simulink model "LADRC_Control"  (R2022a)
settings: Solver=VariableStepAuto  StartTime=0.0  StopTime=20  RelTol=1e-3
undefined symbols (not defined in the file or in its folder): b1, b2, wc, wo
libraries: slpidlib x1
settings Model: Creator=45489  LastModifiedBy=45489
settings SolverCC: AlgebraicLoopSolver=TrustRegion
settings DebuggingCC: UnconnectedInputMsg=warning  UnconnectedOutputMsg=warning  UnconnectedLineMsg=warning  SFMachineParentedDataDiag=warning

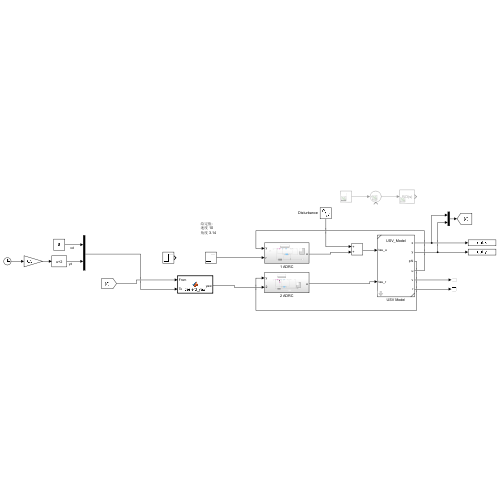
[thumbnail: Simulink's stored preview of the top-level diagram]
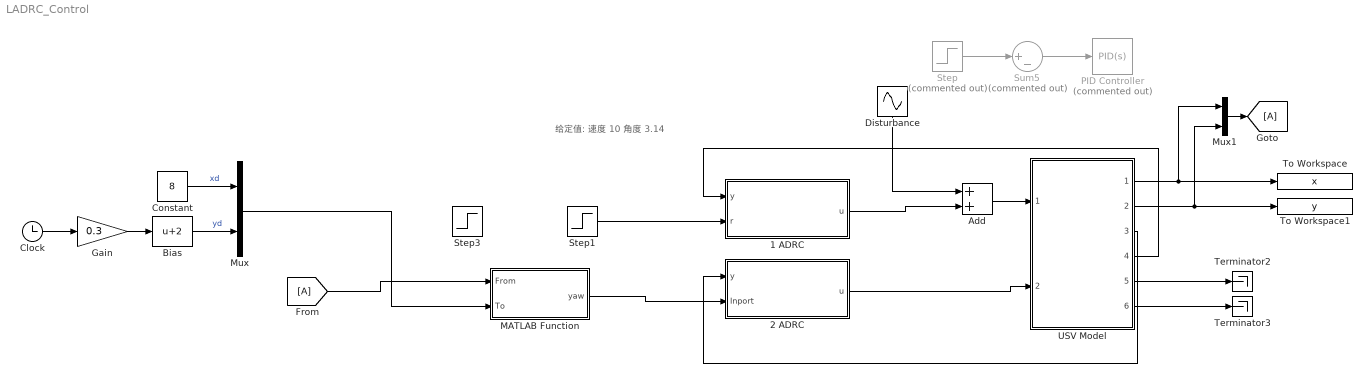
== system LADRC_Control ==
  note: 给定值:
      | 速度 10
      | 角度 3.14
  1 ADRC : Subsystem
  2 ADRC : Subsystem
  Add : Sum
  Bias : Bias  Bias=2  SaturateOnIntegerOverflow=off
  Clock : Clock
  Constant : Constant  Value=8
  Disturbance : Sin  Amplitude=5  Bias=1  SampleTime=0
  From : From
  Gain : Gain  Gain=0.3
  Goto : Goto
  MATLAB Function : MATLAB Function  TreatAsAtomicUnit=on
  Mux : Mux  Inputs=2
  Mux1 : Mux  Inputs=2
  PID Controller : slpidlib/PID Controller  Commented=on  Controller=PID  Form=Parallel  TimeDomain=Continuous-time  UseExternalTs=off  SampleTime=-1  IntegratorMethod=Forward Euler  FilterMethod=Forward Euler  ControllerParametersSource=internal  P=2  I=0  UseKiTs=off  D=1  N=100  UseFilter=on  TunerSelectOption=Transfer Function Based (PID Tuner App)  InitialConditionSource=internal  InitialConditionForIntegrator=0  InitialConditionForFilter=0  DifferentiatorICPrevScaledInput=0  ExternalReset=none  TrackingMode=off  Kt=1  LimitOutput=off  SatLimitsSource=internal  UpperSaturationLimit=inf  LowerSaturationLimit=-inf  LinearizeAsGain=on  AntiWindupMode=none  Kb=1  POutMin=[]  POutMax=[]  IOutMin=[]  IOutMax=[]  DOutMin=[]  DOutMax=[]  NOutMin=[]  NOutMax=[]  SumOutMin=[]  SumOutMax=[]  SaturationOutMin=[]  SaturationOutMax=[]  PParamMin=[]  PParamMax=[]  IParamMin=[]  IParamMax=[]  DParamMin=[]  DParamMax=[]  NParamMin=[]  NParamMax=[]  KbParamMin=[]  KbParamMax=[]  KtParamMin=[]  KtParamMax=[]  KbOutMin=[]  KbOutMax=[]  KtOutMin=[]  KtOutMax=[]  IntegratorOutMin=[]  IntegratorOutMax=[]  FilterOutMin=[]  FilterOutMax=[]  SumI1OutMin=[]  SumI1OutMax=[]  SumI2OutMin=[]  SumI2OutMax=[]  SumI3OutMin=[]  SumI3OutMax=[]  SumI4OutMin=[]  SumI4OutMax=[]  SumDOutMin=[]  SumDOutMax=[]  DifferentiatorOutMin=[]  DifferentiatorOutMax=[]  FilterDiffOutCoefMin=[]  FilterDiffOutCoefMax=[]  ReciprocalOutMin=[]  ReciprocalOutMax=[]  SumDenOutMin=[]  SumDenOutMax=[]  SumNumOutMin=[]  SumNumOutMax=[]  DivideOutMin=[]  DivideOutMax=[]  UdiffTsProdOutMin=[]  UdiffTsProdOutMax=[]  NTsProdOutMin=[]  NTsProdOutMax=[]  UintegralTsProdOutMin=[]  UintegralTsProdOutMax=[]  UngainTsProdOutMin=[]  UngainTsProdOutMax=[]  IntegratorContinuousStateAttributes=''  IntegratorStateMustResolveToSignalObject=off  IntegratorRTWStateStorageClass=Auto  FilterContinuousStateAttributes=''  FilterStateMustResolveToSignalObject=off  FilterRTWStateStorageClass=Auto  ParallelPVariant=InternalParameters  IdealPVariant=Disabled  IVariant=InternalParameters  DVariant=InternalParameters  IntegratorVariant=Continuous  SatVariant=Disabled  AWVariant=Passthrough  PCopyVariant=Disabled  TRVariant=Disabled  FdbkBlocksVariant=Forward  IdealPFdbkVariant=Disabled  SatFdbkVariant=Disabled  DerivativeFilterVariant=ContFilter  NVariant=InternalParameters  NCopyVariant=Disabled  FilterICVariant=InternalICsFilter  IntegratorICVariant=InternalICs  ExternalResetVariant=Disabled  TRSumVariant=Passthrough  SumFdbkVariant=Disabled  SumVariant=Sum_PID  TsampFilterVariant=InternalTs  TsampNgainVariant=Passthrough  TsampIntegralVariant=Passthrough  ExternalSaturationOutDataTypeStr=Inherit: Same as second input  aMode=0
  Step : Step  Commented=on  Time=1.52  After=3.14  SampleTime=0
  Step1 : Step  After=0.3  SampleTime=0
  Step3 : Step  After=0.3  SampleTime=0
  Sum5 : Sum  Commented=on  Inputs=|+-
  Terminator2 : Terminator
  Terminator3 : Terminator
  To Workspace : ToWorkspace  VariableName=x  SaveFormat=Timeseries  SampleTime=-1
  To Workspace1 : ToWorkspace  VariableName=y  SaveFormat=Timeseries  SampleTime=-1
  USV Model : Subsystem  ReferencedSubsystem=USV_Model  x=init_x  y=init_y  psi=init_psi
  wires:
  USV Model/3 -> 2 ADRC/1(y)
  2 ADRC/1(u) -> USV Model/2
  Sum5/1 -> PID Controller/1
  1 ADRC/1(u) -> Add/2
  Step/1 -> Sum5/1
  USV Model/4 -> 1 ADRC/1(y)
  USV Model/1 -> Mux1/1, To Workspace/1
  USV Model/2 -> Mux1/2, To Workspace1/1
  USV Model/5 -> Terminator2/1
  Add/1 -> USV Model/1
  USV Model/6 -> Terminator3/1
  Disturbance/1 -> Add/1
  Step1/1 -> 1 ADRC/2(r)
  Gain/1 -> Bias/1
  Bias/1 -> Mux/2  "yd"
  MATLAB Function/1(yaw) -> 2 ADRC/2(Inport)
  From/1 -> MATLAB Function/1(From)
  Constant/1 -> Mux/1  "xd"
  Mux/1 -> MATLAB Function/2(To)
  Clock/1 -> Gain/1
  Mux1/1 -> Goto/1

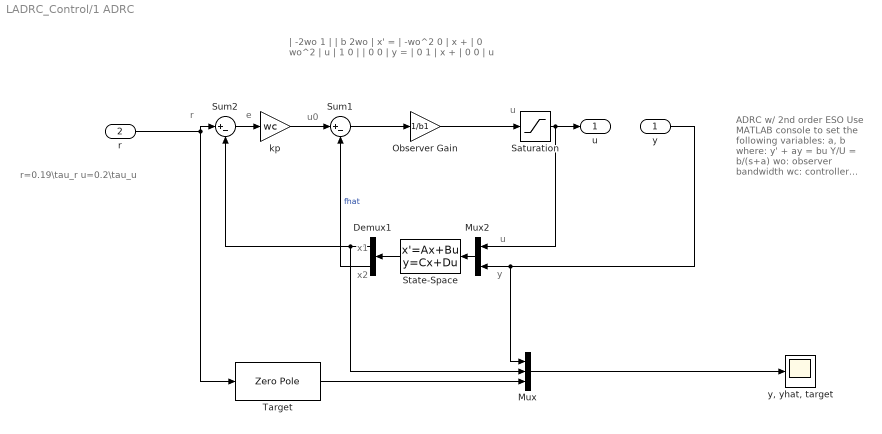
== system LADRC_Control/1 ADRC ==
  note: r=0.19\tau_r
      |
      | u=0.2\tau_u
  note: y
  note: u0
  note: e
  note: r
  note: x1
  note: u
  note: x2
  note: | -2wo  1 |     | b 2wo  |
      | x' = | -wo^2 0 | x + | 0 wo^2 | u
      |
      |      | 1 0 |     | 0 0 |
      | y  = | 0 1 | x + | 0 0 | u
  note: u
  note: ADRC w/ 2nd order ESO
      |
      | Use MATLAB console
      | to set the following
      | variables:
      |
      | a, b where:
      | y' + ay = bu
      | Y/U = b/(s+a)
      |
      | wo: observer bandwidth
      | wc: controller bandwidth
  y : Inport
  r : Inport  Port=2
  Demux1 : Demux  Outputs=2
  Mux : Mux  Inputs=3
  Mux2 : Mux  Inputs=2
  Observer Gain : Gain  Gain=1/b1
  Saturation : Saturate  UpperLimit=100  LowerLimit=0
  State-Space : StateSpace  A=[-2*wo 1;-wo^2 0]  B=[b1 2*wo; 0 wo^2]  C=eye(2)  D=zeros(2,2)  InitialCondition=0
  Sum1 : Sum  Inputs=|+-
  Sum2 : Sum  Inputs=|+-
  Target : ZeroPole  Zeros=[]  Poles=[-wc]  Gain=[wc]
  kp : Gain  Gain=wc
  "y, yhat, target" : Scope
  u : Outport
  wires:
  Mux2/1 -> State-Space/1
  Demux1/2 -> Sum1/2  "fhat"
  State-Space/1 -> Demux1/1
  Demux1/1 -> Sum2/2, Mux/2
  Observer Gain/1 -> Saturation/1
  Mux/1 -> "y, yhat, target"/1
  kp/1 -> Sum1/1
  Sum2/1 -> kp/1
  Sum1/1 -> Observer Gain/1
  y/1 -> Mux2/2, Mux/1
  r/1 -> Sum2/1, Target/1
  Target/1 -> Mux/3
  Saturation/1 -> Mux2/1, u/1

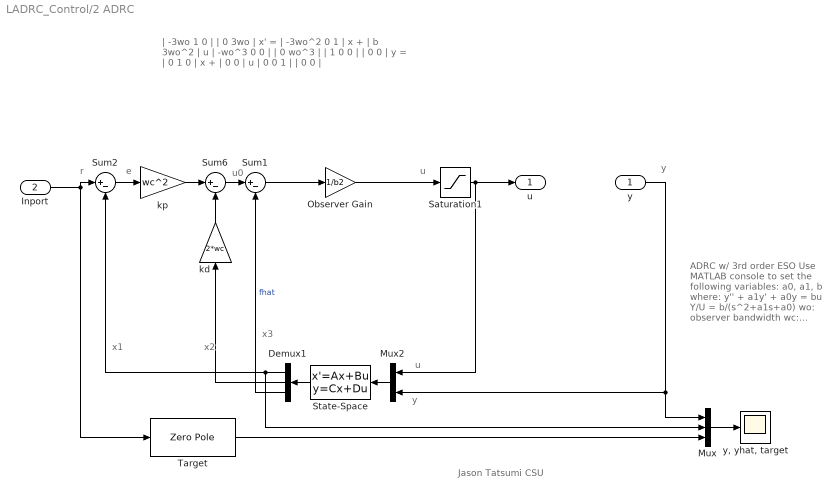
== system LADRC_Control/2 ADRC ==
  note: y
  note: Jason Tatsumi
      | CSU
  note: y
  note: u
  note: u
  note: x1
  note: x2
  note: x3
  note: ADRC w/ 3rd order ESO
      |
      | Use MATLAB console
      | to set the following
      | variables:
      |
      | a0, a1,  b where:
      | y'' + a1y' + a0y = bu
      | Y/U = b/(s^2+a1s+a0)
      |
      | wo: observer bandwidth
      | wc: controller bandwidth
  note: u0
  note: r
  note: e
  note: | -3wo   1 0 |     | 0 3wo   |
      | x' = | -3wo^2 0 1 | x + | b 3wo^2 | u
      |      | -wo^3  0 0 |     | 0 wo^3  |
      |
      |      | 1 0 0 |     | 0 0 |
      | y  = | 0 1 0 | x + | 0 0 | u
      |      | 0 0 1 |     | 0 0 |
  y : Inport
  Inport : Inport  Port=2
  Demux1 : Demux  Outputs=3
  Mux : Mux  Inputs=3
  Mux2 : Mux  Inputs=2
  Observer Gain : Gain  Gain=1/b2
  Saturation1 : Saturate  UpperLimit=+50  LowerLimit=-50
  State-Space : StateSpace  A=[-3*wo 1 0;-3*wo^2 0 1;-wo^3 0 0]  B=[0 3*wo;b2 3*wo^2 ; 0 wo^3 ]  C=eye(3)  D=zeros(3,2)  InitialCondition=0
  Sum1 : Sum  Inputs=|+-
  Sum2 : Sum  Inputs=|+-
  Sum6 : Sum  Inputs=|+-
  Target : ZeroPole  Zeros=[]  Poles=[-wc -wc]  Gain=[wc^2]
  kd : Gain  Gain=2*wc
  kp : Gain  Gain=wc^2
  "y, yhat, target" : Scope
  u : Outport
  wires:
  State-Space/1 -> Demux1/1
  kd/1 -> Sum6/2
  y/1 -> Mux2/2, Mux/1
  Target/1 -> Mux/3
  Mux2/1 -> State-Space/1
  Demux1/2 -> kd/1
  Sum6/1 -> Sum1/1
  Demux1/3 -> Sum1/2  "fhat"
  kp/1 -> Sum6/1
  Inport/1 -> Sum2/1, Target/1
  Mux/1 -> "y, yhat, target"/1
  Observer Gain/1 -> Saturation1/1
  Demux1/1 -> Sum2/2, Mux/2
  Sum1/1 -> Observer Gain/1
  Sum2/1 -> kp/1
  Saturation1/1 -> Mux2/1, u/1

== matlab function LADRC_Control/MATLAB Function ==
  data: From input; yaw output; To input
function yaw = desierd_yaw(From, To)
% generate path
% t=[0:0.1:30];
% x=8*ones(size(t));
% y=t+2;
% horzcat(x',y')

% closest point


% calculate yaw
d=To-From;
yaw=0;
if d(1)>0
    yaw=atan(d(2)/d(1));
elseif d(1)<=0 && d(2) >0
    yaw=pi+atan(d(2)/d(1));
elseif d(1)<=0 && d(2)<=0
    yaw=-pi+atan(d(2)/d(1));
end
